simulink model "ctrl_student_HIL_copy2"  (R2015a)
settings: Solver=ode3  StartTime=0.0  StopTime=inf  RelTol=1e-3
libraries: dspstat3 x1, simulink x1
(part 3 of 3)

== matlab function ctrl_student_HIL_copy2/joystick/Contoller_Map ==
  data: current_mode input; PosXLeft input; PosYLeft input; R2 input; tau_x output; tau_y output; tau_yaw output; glob_forces input
function [tau_x,tau_y,tau_yaw] = fcn(current_mode,PosXLeft,PosYLeft,R2,glob_forces)

if current_mode==2
    tau_x=-PosYLeft*glob_forces(1);
    tau_y=0;
    tau_yaw=PosXLeft*glob_forces(3); 
else
    tau_x=-PosYLeft*glob_forces(1);
    tau_y=PosXLeft*glob_forces(2);
    tau_yaw=R2*glob_forces(3);
end

end

== matlab function ctrl_student_HIL_copy2/joystick/Force Allocation ==
  data: current_mode input; tau_x input; f_vspx output; tau_y input; tau_yaw input; f_vspy output; f_bt output
function [f_vspx,f_vspy,f_bt] = fcn(current_mode,tau_x,tau_y,tau_yaw)
l_bt=0.3875;
l_vsp=-0.4575;

if current_mode==2
    f_vspx=tau_x;
    f_vspy=0;
    f_bt=tau_y;
else
    %new equations from Silas 31/1/2017, based on Matlab inversion of B matrix
    f_vspx=tau_x;
    f_vspy=(l_bt*tau_y)/(l_bt - l_vsp) - tau_yaw/(l_bt - l_vsp);
    f_bt=tau_yaw/(l_bt - l_vsp) - (l_vsp*tau_y)/(l_bt - l_vsp);
end

%original equations from 30/1/2017
% f_vspx=tau_x;
% f_vspy=(tau_yaw-tau_y*l_bt)/(l_vsp-l_bt);
% f_bt=tau_y-f_vspy;

%tau_yaw = f_vspy*l_vsp+f_bt*l_bt
%tau_y=f_vspy+f_bt
%solve for f_bt and f_vspy




end

== matlab function ctrl_student_HIL_copy2/Noise generator/Downsample	signal/MATLAB Function ==
  data: f input; h input; i input; count output
function count = fcn(f,h,i)
%#codegen
sampling_time = 1/f;
if (i+1)*h >= sampling_time
    count = 0;
else
    count = i+1;
end

== matlab function ctrl_student_HIL_copy2/joystick/Force2Control ==
  data: f_vspx input; u_vsp output; f_vspy input; f_bt input; alpha output; u_bt output; sat_forces input
function [u_vsp,alpha,u_bt]   = fcn(f_vspx,f_vspy,f_bt,sat_forces)

u_vsp=sqrt(f_vspx^2+f_vspy^2)/sat_forces(1);
u_bt=f_bt/sat_forces(2);
alpha=atan2(f_vspy,f_vspx); 


end

== matlab function ctrl_student_HIL_copy2/Noise generator/Sample & hold/MATLAB Function1 ==
  data: counter input; input input; hold input; output output
function output = fcn(counter,input,hold)
%#codegen

if counter == 0
    output = input;
else
    output = hold;
end

== matlab function ctrl_student_HIL_copy2/joystick/Sat_Chk_BT ==
  data: u_inn input; u_out output; error output
function [u_out, error]= fcn(u_inn)

if u_inn > 1 || u_inn <-1
    u_out=0;
    error=true;
else
    u_out=u_inn;
    error=false;

end

== matlab function ctrl_student_HIL_copy2/joystick/Sat_Chk_VSP ==
  data: u_inn input; u_out output; error output
function [u_out, error]= fcn(u_inn)

if u_inn > 1 || u_inn <-1
    u_out=0;
    error=true;
else
    u_out=u_inn;
    error=false;

end

== matlab function ctrl_student_HIL_copy2/joystick/Sel_Control_Mode ==
  data: previous_condition input; select input; current_mode output
function current_mode= fcn(previous_condition, select)

if select==1
    if previous_condition ==2
        current_mode=3;
    else
        current_mode=2;
    end
else
    current_mode=previous_condition;
end

end

== matlab function ctrl_student_HIL_copy2/kinetics ==
  data: tau input; nu_dot output; nu input
function nu_dot = CSE1_nu_dot(tau,nu)

u   = nu(1);
v   = nu(2);
r   = nu(3);

tau = [tau(1);tau(2);tau(3)];
%% MATRICES

m    = 14.79;   I_z  =  1.7600;   x_g = 0.0375;       % x_g  =  0.0460; % Table B.1


%% Added mass
X_ud  =     -2.0;											% Table B.1
					Y_vd =     -1.0;	N_vd =    -0.0;		% Table B.1 guestimate
					Y_rd =      -0.0;	N_rd =    -1.0;		% Table B.1

%% Total mass matrix
m_11 = m-X_ud;
m_22 = m-Y_vd;
m_23 = m*x_g-Y_rd;
m_32 = m*x_g-N_vd;
m_33 = I_z-N_rd;

M    = [m_11 0    0
        0    m_22 m_23
        0    m_32 m_33];
	
%% Damping coefficients
% Comments at the end of the lines indicate the old values used.
X_u		= -0.6555;		X_v		= 0;
X_uu 	= 0.3545;		X_vv	= -2.443;
X_uuu 	= -3.787;		X_vvv	= 0;

						Y_v		= -1.33; 			Y_r		= -7.250; % Y_r
						Y_vv	= -2.776;			Y_rr	= -3.450; % Y_rr
						Y_vvv	= -64.91;			Y_rrr	= 0;
						
						Y_rv	= -0.805;			Y_vr	= -0.845; % Y_rv, Y_vr

						N_v		= 0;				N_r		= -1.900; % N_r
						N_vv	= -0.2088;			N_rr	= -0.750; % N_rr
						N_vvv	= 0;				N_rrr	= 0;
						
						N_rv	= 0.130;			N_vr	= 0.080; % N_rv, N_vr

%% Correolis matrix
c_13 = -(m-Y_vd)*v-(m*x_g-Y_rd)*r;
c_23 = (m-X_ud)*u;
C    = [0     0     c_13
        0     0     c_23
        -c_13 -c_23 0   ];

%% Assembly of the damping matrix
d_11 = -X_u - X_uu*abs(u) - X_uuu*u^2;
d_22 = -Y_v - Y_vv*v - Y_vvv*v^2 - Y_rv*abs(r);
d_33 = -N_r - N_rr*abs(r) - N_rrr*r^2 - N_vr*abs(v); % using abs(r)

d_12 = -X_v - X_vv*v - X_vvv*v^2;
d_23 = -Y_r - Y_rr*abs(r) - Y_rrr*r^2 - Y_vr*abs(v);
d_32 = -N_v - N_vv*v - N_vvv*v^2 - N_rv*abs(r);

D    = [d_11 0 0
        0    d_22 d_23
        0    d_32 d_33];



%% CALCULATION
nu_dot = M\(tau-(C+D)*nu);

== matlab function ctrl_student_HIL_copy2/DropOut_detector/dropoutDetect ==
  data: etaPrev input; eta input; dropout output; etaOut output
function [dropout,etaOut]= fcn(etaPrev,eta)

etaTemp=[etaPrev [eta; 0]];

if max(etaTemp(:,4))==1
     dropout=1;
elseif min(eta-etaTemp(1:3,end-1))==0
    dropout=1;
    etaTemp(4,end)=1;
elseif var(etaTemp(1,:))==0 || var(etaTemp(2,:))==0 || var(etaTemp(2,:))==0
    dropout=1;
else
    dropout=0;
end

etaOut=etaTemp(:,2:end);

end

== matlab function ctrl_student_HIL_copy2/safety zone /Safety Act ==
  data: joyStick input; safetySig_1 input; safetySig_2 input; safetySig_3 input; safetySig_4 input; thrust_out output; vel input; switch_sig output
function [thrust_out,switch_sig] = fcn(joyStick,safetySig_1,safetySig_2,safetySig_3,safetySig_4,vel)

switch_sig=0;
thrust_out=zeros(3,1);
K=[1;1];    

    if safetySig_1 == 0 && safetySig_2 == 0 && safetySig_3 == 0 && safetySig_4 == 0   %Check to see if intervention is requiered
        
    switch_sig = 0; %Intervention is NOT requiered
    thrust_out =[0;0;0];
    else
    switch_sig=1;   %Intervention IS requiered
    
        if  safetySig_1==1 || safetySig_2==1 %Problem in X dir
            
            if joyStick(2)==0 %Check if inputforce fore is zero or correct, (but the velocity might not be)
               %Perhaps a proprtional gain depending on the velocity?
               if vel(1)>0 && safetySig_2==1
                   ThrustX=K(1)*-vel(1);
               elseif vel(1)< 0 && safetySig_1==1
                   ThrustX=K(1)*-vel(1);
               else
                ThrustX=K(1)*vel;
               end
                thrust_out=[ThrustX;joyStick(2);joyStick(3)];
            elseif joyStick(2) <0 && safetySig_2==1     %X cord to small, but thrust right way
                thrust_out=[joyStick(1);joyStick(2);joyStick(3)];
            elseif joyStick(2) >0 && safetySig_1==1     %X cord to large, but thrust right way
                thrust_out=[joyStick(1);joyStick(2);joyStick(3)];
            else
            thrust_out=[-joyStick(1);joyStick(2);joyStick(3)];
            end
            
            
        else %Problem in Y dir
            if joyStick(2)==0 %Check if inputforce fore is zero or correct
                %Perhaps a proprtional gain depending on the velocity?  
                if vel(1)>0 && safetySig_2==1
                   ThrustY=K(1)*-vel(1);
               elseif vel(1)< 0 && safetySig_1==1
                   ThrustY=K(1)*-vel(1);
               else
                ThrustY=K(1)*vel;
                end
                thrust_out=[joyStick(1);ThrustY;joyStick(3)];
                
                
            elseif joyStick(2) <0 && safetySig_1==1     %X cord to small
                thrust_out=[joyStick(1);joyStick(2);joyStick(3)];
            elseif joyStick(2) >0 && safetySig_2==1     %X cord to large
                thrust_out=[joyStick(1);joyStick(2);joyStick(3)];
            else
            thrust_out=[joyStick(1);-joyStick(2);joyStick(3)];
            end
        end
    end
                %joyStic is in vector type [X,Y,M]
end

== matlab function ctrl_student_HIL_copy2/safety zone /safety check ==
  data: eta input; safety_sig_1 output; safety_sig_2 output; safety_sig_3 output; safety_sig_4 output; lim input
function [safety_sig_1,safety_sig_2,safety_sig_3,safety_sig_4]= fcn(eta,lim)


safety_sig=[0;0;0;0];%orginal safety signal
%lim=[40.00;0;6.45;0];%space limitation [x_max;x_min;y_max;y_min]
if eta(1)>=lim(1)
    safety_sig_1 = 1;
    safety_sig_2= 0;
elseif eta(1)<=lim(2)
    safety_sig_2 = 1;
    safety_sig_1=0;
else
    safety_sig_1 = 0;
    safety_sig_2 = 0;
end
if eta(2)>lim(3)
    safety_sig(3) = 1;
elseif eta(2)<lim(4)
    safety_sig(4) = 1;
else
    safety_sig(3) = 0;
    safety_sig(4) = 0;
end
% safety_sig_1=safety_sig(1);
% safety_sig_2=safety_sig(2);
safety_sig_3=safety_sig(3);
safety_sig_4=safety_sig(4);

end

== matlab function ctrl_student_HIL_copy2/Dropout_simulator/MATLAB Function ==
  data: X_in input; X_out output; Y_out output; Yaw_out output; Y_in input; Yaw_in input; Dropoutsignal input; X_prev input; Y_prev input; Yaw_prev input
function [X_out,Y_out,Yaw_out] = fcn(X_in,Y_in,Yaw_in,Dropoutsignal,X_prev,Y_prev,Yaw_prev)
X_out=-1;
Y_out=-1;
Yaw_out=-1;


switch Dropoutsignal
    case 0
        X_out =X_in;
        Y_out=Y_in;
        Yaw_out=Yaw_in;
        
    case 1        
        X_out =X_prev;
        Y_out=Y_prev;
        Yaw_out=Yaw_prev;
end


end

== matlab function ctrl_student_HIL_copy2/DropoutAction/accInjection ==
  data: uLast input; dropout input; uIn input; u_hat output; dVel input
function u_hat=accInj(uLast,dropout,uIn,dVel)

if dropout==false
    u_hat=uIn;
else
    u_hat=uLast+dVel;
end
